simulink model "Steuerung_A2_Final"  (R2018a)
settings: Solver=ode1  StartTime=0.0  StopTime=inf  FixedStep=1/10  RelTol=1e-3  EnableMultiTasking=on
undefined symbols (not defined in the file or in its folder): gray
libraries: simulink x4, PiCar_library x1, visiontextngfix x1, embdlinuxlib x1
settings Model: SimulationMode=external  Creator=raspberry  LastModifiedBy=Kevin
settings SolverCC: PositivePriorityOrder=on
settings OptimizationCC: PassReuseOutputArgsAs=Individual arguments  MaxStackSize=64
settings DebuggingCC: ParameterTunabilityLossMsg=error
settings HardwareCC: ProdBitPerPointer=32  ProdBitPerSizeT=32  ProdBitPerPtrDiffT=32  ProdLargestAtomicInteger=Long  ProdLargestAtomicFloat=Double  ProdWordSize=32  ProdHWDeviceType=ARM Compatible->ARM Cortex
settings RTWCC: SystemTargetFile=ert.tlc  HardwareBoard=Raspberry Pi  TLCOptions="-aInlineSetEventsForThisBaseRateFcn=TLC_FALSE -aSuppressMultiTaskScheduler=TLC_FALSE  -aRateBasedStepFcn=0"  TemplateMakefile=ert_default_tmf  Toolchain=GNU GCC Raspberry Pi
settings RTWCC: CustomTerminator=|
  | /* Send ALL_LED_OFF Signal to all PWM driver chip address
  | See PCA9685 user manual, section 7.3.4
  | Set Chip in sleep mode, section 7.3.1
  | Reset the PWM ON/OFF states for all LEDs */
  | 
  | int fd;
  | 
  | fd = wiringPiI2CSetup(0x70);
  | wiringPiI2CWriteReg8(fd, 0x00, 0x11); // sleep mode
  | wiringPiI2CWriteReg8(fd, 0xFD, 0x10); // all LED off
  | wiringPiI2CWriteReg8(fd, 0xFC, 0x00);
  | wiringPiI2CWriteReg8(fd, 0xFB, 0x00);
  | wiringPiI2CWriteReg8(fd, 0xFA, 0x00);
settings CodeAppCC: ForceParamTrailComments=on  IgnoreCustomStorageClasses=off  OperatorAnnotations=on  SimulinkDataObjDesc=on  SFDataObjDesc=on  MATLABFcnDesc=on  InsertBlockDesc=on  StateflowObjectComments=on  MATLABSourceComments=on
settings ERTTargetCC: SupportVariableSizeSignals=on  ExtMode=on  ExtModeMexArgs='192.168.4.1' 0 17725

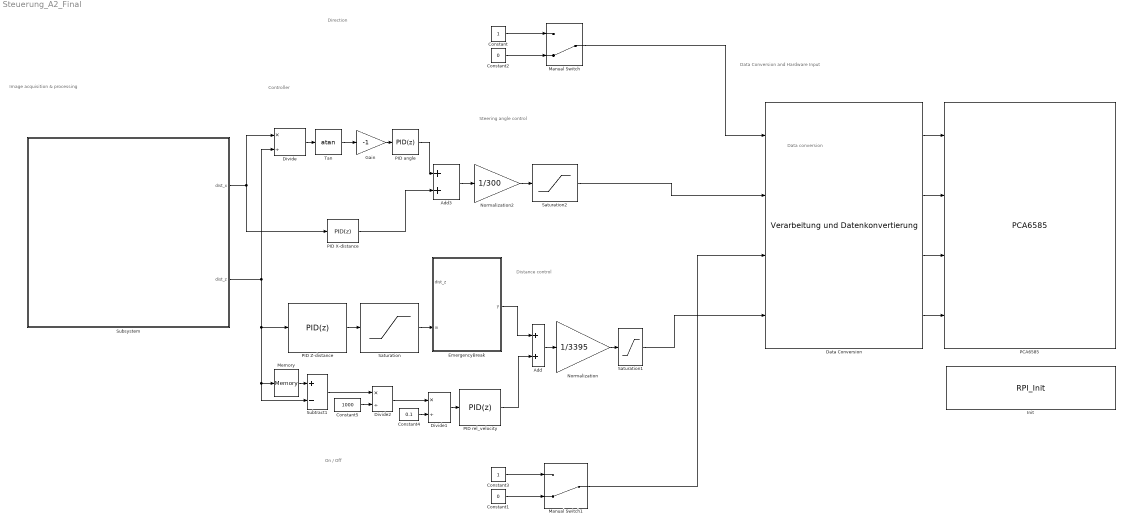
== system Steuerung_A2_Final ==
  note: Steering angle control
  note: Data Conversion and Hardware Input
  note: Data conversion
  note: Direction
  note: On / Off
  note: Image acquisition & processing
  note: Controller
  note: Distance control
  Add : Sum
  Add3 : Sum
  Constant : Constant
  Constant1 : Constant  Value=0
  Constant2 : Constant  Value=0
  Constant3 : Constant
  Constant4 : Constant  Value=0.1
  Constant5 : Constant  Value=1000
  Data Conversion : PiCar_library/Verarbeitung und Datenkonvertierung
      link override Constant3: Value=1160
  Divide : Product  Inputs=*/
  Divide1 : Product  Inputs=*/
  Divide2 : Product  Inputs=*/
  EmergencyBreak : MATLAB Function  TreatAsAtomicUnit=on
  Gain : Gain  Gain=-1
  Init : S-Function  Priority=1  InitFcn=try, set_param(gcb,'FunctionName','RPI_Init'), end  FunctionName=RPI_Init  SFunctionModules=RPI_Init_wrapper  SFunctionDeploymentMode=off  EnableBusSupport=off  mask(S-Function Builder){}
      mask help: Simulink:masks:SFunctionBuilder_MD
      mask init:
      | val = [[.9  0.75 0.75 1 1 .9 .9 1]',[1 1 0.75 0.75 .9 .9 1 .9]'];try , sys = get_param(gcb,'SfunBuilderFcnName');if isempty(sys), sys = get_param(gcb,'FunctionName'); end,catch, sys = get_param(gcb,'FunctionName'); end
      settings: CopyFcn=set_param(gcbh,'LinkStatus','none')  PreSaveFcn=try, set_param(gcb,'FunctionName','RPI_Init'), end  OpenFcn=sfunctionwizard(gcbh)
      mask Display:
      | plot(val(:,1),val(:,2))
      | disp(sys)
  Manual Switch : ManualSwitch  CurrentSetting=0
  Manual Switch1 : ManualSwitch  CurrentSetting=0
  Memory : Memory
  Normalization : Gain  Gain=1/3395
  Normalization2 : Gain  Gain=1/300
  PCA6585 : S-Function  InitFcn=try, set_param(gcb,'FunctionName','PCA6585'), end  FunctionName=PCA6585  SFunctionModules=PCA6585_wrapper  SFunctionDeploymentMode=off  EnableBusSupport=off  mask(S-Function Builder){}
      mask help: Simulink:masks:SFunctionBuilder_MD
      mask init: same as Steuerung_A2_Final/Init
      settings: CopyFcn=set_param(gcbh,'LinkStatus','none')  PreSaveFcn=try, set_param(gcb,'FunctionName','PCA6585'), end  OpenFcn=sfunctionwizard(gcbh)
      mask Display: plot(val(:,1),val(:,2)),disp(sys), port_label('input',1,'IN_1'), port_label('input',2,'IN_2'), port_label('input',3,'PWM'), port_label('input',4,'SERVO')
  PID X-distance : simulink/Continuous/PID Controller  Controller=PID  TimeDomain=Discrete-time  SampleTime=-1  IntegratorMethod=Forward Euler  FilterMethod=Forward Euler  Form=Parallel  UseFilter=on  ControllerParametersSource=internal  P=0.1  I=0  D=0  N=100  InitialConditionSource=internal  InitialConditionForIntegrator=0  InitialConditionForFilter=0  ExternalReset=none  LimitOutput=off  UpperSaturationLimit=inf  LowerSaturationLimit=-inf  LinearizeAsGain=off  AntiWindupMode=none  Kb=1  TrackingMode=off  Kt=1  PParamMin=[]  PParamMax=[]  IParamMin=[]  IParamMax=[]  DParamMin=[]  DParamMax=[]  NParamMin=[]  NParamMax=[]  KbParamMin=[]  KbParamMax=[]  KtParamMin=[]  KtParamMax=[]  POutMin=[]  POutMax=[]  IOutMin=[]  IOutMax=[]  DOutMin=[]  DOutMax=[]  NOutMin=[]  NOutMax=[]  KbOutMin=[]  KbOutMax=[]  KtOutMin=[]  KtOutMax=[]  IntegratorOutMin=[]  IntegratorOutMax=[]  FilterOutMin=[]  FilterOutMax=[]  SumOutMin=[]  SumOutMax=[]  SumI1OutMin=[]  SumI1OutMax=[]  SumI2OutMin=[]  SumI2OutMax=[]  SumI3OutMin=[]  SumI3OutMax=[]  SumDOutMin=[]  SumDOutMax=[]  SaturationOutMin=[]  SaturationOutMax=[]  IntegratorContinuousStateAttributes=''  IntegratorStateMustResolveToSignalObject=off  IntegratorRTWStateStorageClass=Auto  FilterContinuousStateAttributes=''  FilterStateMustResolveToSignalObject=off  FilterRTWStateStorageClass=Auto  DifferentiatorICPrevScaledInput=0  DifferentiatorOutMin=[]  DifferentiatorOutMax=[]  FilterDiffOutCoefMin=[]  FilterDiffOutCoefMax=[]  SumDenOutMin=[]  SumDenOutMax=[]  SumNumOutMin=[]  SumNumOutMax=[]  ReciprocalOutMin=[]  ReciprocalOutMax=[]  DivideOutMin=[]  DivideOutMax=[]  TunerSelectOption=Transfer Function Based (PID Tuner App)
  PID Z-distance : simulink/Continuous/PID Controller  Controller=PID  TimeDomain=Discrete-time  SampleTime=-1  IntegratorMethod=Forward Euler  FilterMethod=Forward Euler  Form=Parallel  UseFilter=on  ControllerParametersSource=internal  P=0.5  I=0.01  D=0  N=100  InitialConditionSource=internal  InitialConditionForIntegrator=0  InitialConditionForFilter=0  ExternalReset=none  LimitOutput=off  UpperSaturationLimit=inf  LowerSaturationLimit=-inf  LinearizeAsGain=off  AntiWindupMode=none  Kb=1  TrackingMode=off  Kt=1  PParamMin=[]  PParamMax=[]  IParamMin=[]  IParamMax=[]  DParamMin=[]  DParamMax=[]  NParamMin=[]  NParamMax=[]  KbParamMin=[]  KbParamMax=[]  KtParamMin=[]  KtParamMax=[]  POutMin=[]  POutMax=[]  IOutMin=[]  IOutMax=[]  DOutMin=[]  DOutMax=[]  NOutMin=[]  NOutMax=[]  KbOutMin=[]  KbOutMax=[]  KtOutMin=[]  KtOutMax=[]  IntegratorOutMin=[]  IntegratorOutMax=[]  FilterOutMin=[]  FilterOutMax=[]  SumOutMin=[]  SumOutMax=[]  SumI1OutMin=[]  SumI1OutMax=[]  SumI2OutMin=[]  SumI2OutMax=[]  SumI3OutMin=[]  SumI3OutMax=[]  SumDOutMin=[]  SumDOutMax=[]  SaturationOutMin=[]  SaturationOutMax=[]  IntegratorContinuousStateAttributes=''  IntegratorStateMustResolveToSignalObject=off  IntegratorRTWStateStorageClass=Auto  FilterContinuousStateAttributes=''  FilterStateMustResolveToSignalObject=off  FilterRTWStateStorageClass=Auto  DifferentiatorICPrevScaledInput=0  DifferentiatorOutMin=[]  DifferentiatorOutMax=[]  FilterDiffOutCoefMin=[]  FilterDiffOutCoefMax=[]  SumDenOutMin=[]  SumDenOutMax=[]  SumNumOutMin=[]  SumNumOutMax=[]  ReciprocalOutMin=[]  ReciprocalOutMax=[]  DivideOutMin=[]  DivideOutMax=[]  TunerSelectOption=Transfer Function Based (PID Tuner App)
  PID angle : simulink/Continuous/PID Controller  Controller=PID  TimeDomain=Discrete-time  SampleTime=-1  IntegratorMethod=Forward Euler  FilterMethod=Forward Euler  Form=Parallel  UseFilter=on  ControllerParametersSource=internal  P=1  I=0  D=0  N=100  InitialConditionSource=internal  InitialConditionForIntegrator=0  InitialConditionForFilter=0  ExternalReset=none  LimitOutput=off  UpperSaturationLimit=inf  LowerSaturationLimit=-inf  LinearizeAsGain=off  AntiWindupMode=none  Kb=1  TrackingMode=off  Kt=1  PParamMin=[]  PParamMax=[]  IParamMin=[]  IParamMax=[]  DParamMin=[]  DParamMax=[]  NParamMin=[]  NParamMax=[]  KbParamMin=[]  KbParamMax=[]  KtParamMin=[]  KtParamMax=[]  POutMin=[]  POutMax=[]  IOutMin=[]  IOutMax=[]  DOutMin=[]  DOutMax=[]  NOutMin=[]  NOutMax=[]  KbOutMin=[]  KbOutMax=[]  KtOutMin=[]  KtOutMax=[]  IntegratorOutMin=[]  IntegratorOutMax=[]  FilterOutMin=[]  FilterOutMax=[]  SumOutMin=[]  SumOutMax=[]  SumI1OutMin=[]  SumI1OutMax=[]  SumI2OutMin=[]  SumI2OutMax=[]  SumI3OutMin=[]  SumI3OutMax=[]  SumDOutMin=[]  SumDOutMax=[]  SaturationOutMin=[]  SaturationOutMax=[]  IntegratorContinuousStateAttributes=''  IntegratorStateMustResolveToSignalObject=off  IntegratorRTWStateStorageClass=Auto  FilterContinuousStateAttributes=''  FilterStateMustResolveToSignalObject=off  FilterRTWStateStorageClass=Auto  DifferentiatorICPrevScaledInput=0  DifferentiatorOutMin=[]  DifferentiatorOutMax=[]  FilterDiffOutCoefMin=[]  FilterDiffOutCoefMax=[]  SumDenOutMin=[]  SumDenOutMax=[]  SumNumOutMin=[]  SumNumOutMax=[]  ReciprocalOutMin=[]  ReciprocalOutMax=[]  DivideOutMin=[]  DivideOutMax=[]  TunerSelectOption=Transfer Function Based (PID Tuner App)
  PID rel_velocity : simulink/Continuous/PID Controller  Controller=PID  TimeDomain=Discrete-time  SampleTime=-1  IntegratorMethod=Forward Euler  FilterMethod=Forward Euler  Form=Parallel  UseFilter=on  ControllerParametersSource=internal  P=10  I=0  D=0  N=100  InitialConditionSource=internal  InitialConditionForIntegrator=0  InitialConditionForFilter=0  ExternalReset=none  LimitOutput=off  UpperSaturationLimit=inf  LowerSaturationLimit=-inf  LinearizeAsGain=off  AntiWindupMode=none  Kb=1  TrackingMode=off  Kt=1  PParamMin=[]  PParamMax=[]  IParamMin=[]  IParamMax=[]  DParamMin=[]  DParamMax=[]  NParamMin=[]  NParamMax=[]  KbParamMin=[]  KbParamMax=[]  KtParamMin=[]  KtParamMax=[]  POutMin=[]  POutMax=[]  IOutMin=[]  IOutMax=[]  DOutMin=[]  DOutMax=[]  NOutMin=[]  NOutMax=[]  KbOutMin=[]  KbOutMax=[]  KtOutMin=[]  KtOutMax=[]  IntegratorOutMin=[]  IntegratorOutMax=[]  FilterOutMin=[]  FilterOutMax=[]  SumOutMin=[]  SumOutMax=[]  SumI1OutMin=[]  SumI1OutMax=[]  SumI2OutMin=[]  SumI2OutMax=[]  SumI3OutMin=[]  SumI3OutMax=[]  SumDOutMin=[]  SumDOutMax=[]  SaturationOutMin=[]  SaturationOutMax=[]  IntegratorContinuousStateAttributes=''  IntegratorStateMustResolveToSignalObject=off  IntegratorRTWStateStorageClass=Auto  FilterContinuousStateAttributes=''  FilterStateMustResolveToSignalObject=off  FilterRTWStateStorageClass=Auto  DifferentiatorICPrevScaledInput=0  DifferentiatorOutMin=[]  DifferentiatorOutMax=[]  FilterDiffOutCoefMin=[]  FilterDiffOutCoefMax=[]  SumDenOutMin=[]  SumDenOutMax=[]  SumNumOutMin=[]  SumNumOutMax=[]  ReciprocalOutMin=[]  ReciprocalOutMax=[]  DivideOutMin=[]  DivideOutMax=[]  TunerSelectOption=Transfer Function Based (PID Tuner App)
  Saturation : Saturate  UpperLimit=3400  LowerLimit=-600
  Saturation1 : Saturate  UpperLimit=1  LowerLimit=-1
  Saturation2 : Saturate  UpperLimit=1  LowerLimit=-1
  Subsystem : Subsystem
  Subtract1 : Sum  Inputs=+-
  Tan : Trigonometry  Operator=atan
  wires:
  Constant/1 -> Manual Switch/1
  Constant2/1 -> Manual Switch/2
  Manual Switch/1 -> Data Conversion/1
  Manual Switch1/1 -> Data Conversion/3
  Data Conversion/1 -> PCA6585/1
  Data Conversion/2 -> PCA6585/2
  Data Conversion/3 -> PCA6585/3
  Data Conversion/4 -> PCA6585/4
  Subsystem/2(dist_z) -> PID Z-distance/1, Subtract1/2, Memory/1, Divide/2
  Subsystem/1(dist_x) -> PID X-distance/1, Divide/1
  Tan/1 -> Gain/1
  Divide/1 -> Tan/1
  PID angle/1 -> Add3/1
  PID X-distance/1 -> Add3/2
  Add3/1 -> Normalization2/1
  Normalization2/1 -> Saturation2/1
  Gain/1 -> PID angle/1
  Saturation2/1 -> Data Conversion/2
  Constant3/1 -> Manual Switch1/1
  Constant1/1 -> Manual Switch1/2
  Normalization/1 -> Saturation1/1
  Subtract1/1 -> Divide2/1
  Divide1/1 -> PID rel_velocity/1
  PID Z-distance/1 -> Saturation/1
  Divide2/1 -> Divide1/1
  Constant4/1 -> Divide1/2
  Memory/1 -> Subtract1/1
  Add/1 -> Normalization/1
  Saturation1/1 -> Data Conversion/4
  PID rel_velocity/1 -> Add/2
  EmergencyBreak/1(y) -> Add/1
  Constant5/1 -> Divide2/2
  Saturation/1 -> EmergencyBreak/2(in)

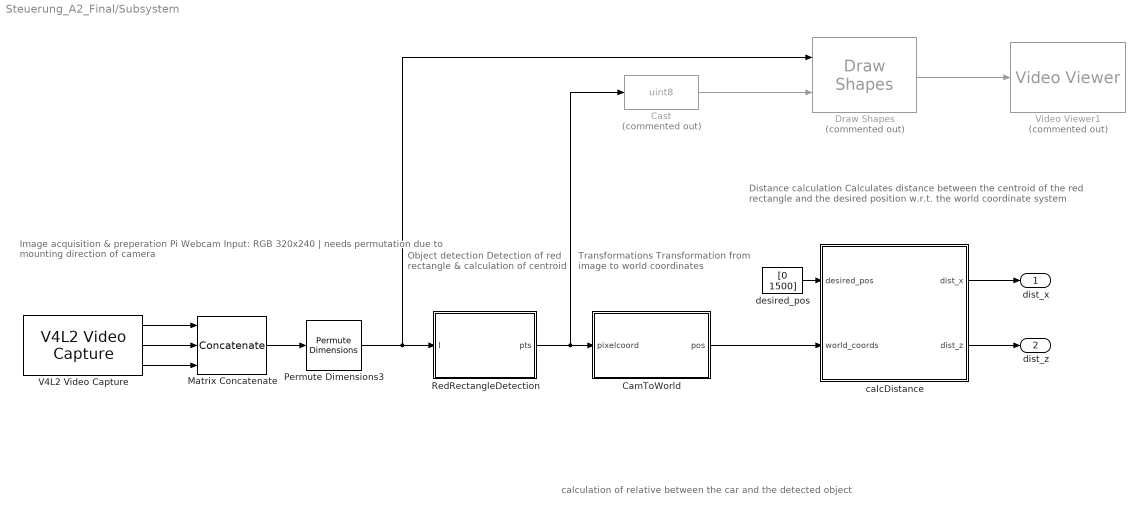
== system Steuerung_A2_Final/Subsystem ==
  note: calculation of relative between the car and the detected object
  note: Object detection
      |
      | Detection of red rectangle &
      | calculation of centroid
  note: Image acquisition & preperation
      |
      | Pi Webcam Input: RGB 320x240 | needs permutation
      | due to mounting direction of camera
  note: Transformations
      |
      | Transformation from image
      | to world coordinates
  note: Distance calculation
      |
      | Calculates distance between the centroid of the red rectangle
      | and the desired position w.r.t. the world coordinate system
  CamToWorld : MATLAB Function  TreatAsAtomicUnit=on
  Cast : DataTypeConversion  Commented=on  OutDataTypeStr=uint8
  Draw Shapes : visiontextngfix/Draw Shapes  Commented=on  shape=Circles  fill=off  lineWidth=1  fillClrSource=Specify via dialog  display=User-specified value  intensity=200  color=[0 0 255]  opacity=0.6  viewport=Entire image  antialiasing=on  inType=Obsolete  imagePorts=One multidimensional signal  prodOutputMode=Binary point scaling  prodOutputWordLength=32  prodOutputFracLength=14  memoryMode=Specify word length  memoryWordLength=16  memoryFracLength=14  roundingMode=Floor  overflowMode=off
      settings: SourceProductName=Computer Vision System Toolbox
  Matrix Concatenate : Concatenate  NumInputs=3  Mode=Multidimensional array  ConcatenateDimension=3
  Permute Dimensions3 : PermuteDimensions  Order=[2,1,3]
  RedRectangleDetection : MATLAB Function  TreatAsAtomicUnit=on
  V4L2 Video Capture : embdlinuxlib/V4L2 Video Capture  m_devName='/dev/video0'  roi=[0, 0, 640, 480]  imSizeSelection=320x240  imSize=[640, 480]  pixelFormat=RGB  pixelOrder=Planar  sampleTime=1/10  simOutput=Colorbars  blockPlatform=Raspberry Pi
      settings: SourceProductName=Simulink Support Package for Raspberry Pi Hardware  SourceProductBaseCode=RASPPI
  Video Viewer1 : VideoViewer  Commented=on  colormapValue=gray(256)  FigPos=[1065 1037 855 929]
  "calcDistance " : MATLAB Function  TreatAsAtomicUnit=on
  desired_pos : Constant  Value=[0 1500]
  dist_x : Outport
  dist_z : Outport  Port=2
  wires:
  "calcDistance "/1(dist_x) -> dist_x/1
  Cast/1 -> Draw Shapes/2
  Draw Shapes/1 -> Video Viewer1/1
  RedRectangleDetection/1(pts) -> Cast/1, CamToWorld/1(pixelcoord)
  CamToWorld/1(pos) -> "calcDistance "/2(world_coords)
  desired_pos/1 -> "calcDistance "/1(desired_pos)
  "calcDistance "/2(dist_z) -> dist_z/1
  Matrix Concatenate/1 -> Permute Dimensions3/1
  V4L2 Video Capture/1 -> Matrix Concatenate/1
  V4L2 Video Capture/2 -> Matrix Concatenate/2
  V4L2 Video Capture/3 -> Matrix Concatenate/3
  Permute Dimensions3/1 -> Draw Shapes/1, RedRectangleDetection/1(I)

== matlab function Steuerung_A2_Final/Subsystem/RedRectangleDetection ==
  data: I input; pts output
function pts  = objectDet  (I)


red = I(:,:,1);
green = I(:,:,2);
blue = I(:,:,3);

red2 = double(red);
green2 = double(green);
blue2 = double(blue);
%out = red > 200 & red < 250 & green > 40 & green < 150 & blue > 90 & blue < 200;

%out = red > 115 & red < 160 & green > 25 & green < 55 & blue > 15 & blue < 40;
out = (100*red2) > (50 * (red2 + green2 + blue2)) & (red2 + green2 + blue2) > 120;



centr = regionprops(out,'centroid');
area = regionprops(out,'area');

area2 = struct2cell(area);
max = 0;
idx = 0;
for i = 1:1:length(area2)
if area2{1,i} > max
max = area2{1,i};
idx = i;
end
end
if max == 0
y1 = length(red(:,1))/2;
x1 = length(red(1,:))/2;
else
help = struct2cell(centr(idx));
x1 = help{1,1}(1);
y1 = help{1,1}(2);
end
pts = [x1,y1,1];
end

== matlab function Steuerung_A2_Final/Subsystem/CamToWorld ==
  data: pixelcoord input; pos output
%CamToWorld([0;0], 10/180*pi, 150, 5);
%alpha in grad
function pos  = CamToWorld(pixelcoord)
plane_height = 72;  %77 bei Iske Buch
alpha = 18.5; %18.5
h= 275 - plane_height;
f_px =[276.3065;275.7723];
image_size = [320;240];
camera_pos = [0;275;-315];

%Pixelkoordinatensystem verschieben
pixelcoord(1) = pixelcoord(1) - image_size(1)/2;
pixelcoord(2) = -pixelcoord(2) + image_size(2)/2;

%Position sch?tzen
alpha = alpha * pi / 180;
z_est = h/cos(alpha) / (tan(alpha) - pixelcoord(2)/f_px(2));
y_est = z_est * pixelcoord(2)/f_px(2);
x_est = z_est * pixelcoord(1)/f_px(1);

%rotieren
pos1 = [1 0 0; 0 cos(alpha) -sin(alpha); 0 sin(alpha) cos(alpha)] * [x_est; y_est; z_est];

%Position der Kamera einbeziehen
pos = pos1 + camera_pos;


end

== matlab function Steuerung_A2_Final/Subsystem/calcDistance  ==
  data: desired_pos input; world_coords input; dist_x output; dist_z output
function [dist_x,dist_z] = calcDistance(desired_pos,world_coords)

dist_x = world_coords(1) - desired_pos(1)-30;  % dist from the centre of the image, for steering
dist_z = world_coords(3) - desired_pos(2);  % dist from the car

% if (dist_z > 0)
%     speed = 100;
% else
%     speed = -600;
% end   
end

== matlab function Steuerung_A2_Final/EmergencyBreak ==
  data: dist_z input; y output; in input
function y = emergencyBrake(dist_z,in)

if dist_z >= -500
    y = in;
else 
    y = -600;
end

end
